simulink model "SimulationLoopNew"  (R2025b)
settings: Solver=VariableStepAuto  StartTime=0.0  StopTime=90  RelTol=1e-3
values from neighbouring files (symbols this model uses):
  dt = 40/10000    (= 0.004)    [constants.m]
  F = StateTransitionMat(z(1:3), z(4:6), R_b2i)    [EstimateStateFCN.m]
  q = q / norm(q)    [EstimateStateFCN.m]
undefined symbols (not defined in the file or in its folder): Checkpoints, constantsASTRA, DiscIntNeverNeededParam, distMode, dt_SIM, HoldTimeReqs, IMU_Rate, K, Light, MIL, u0, x0
libraries: simulink x2, aerolibnav x2, aerolibwind2 x1, dspstat3 x1
settings Model: SimulationMode=accelerator  PacingRate=5  Creator=antho  LastModifiedBy=andrew

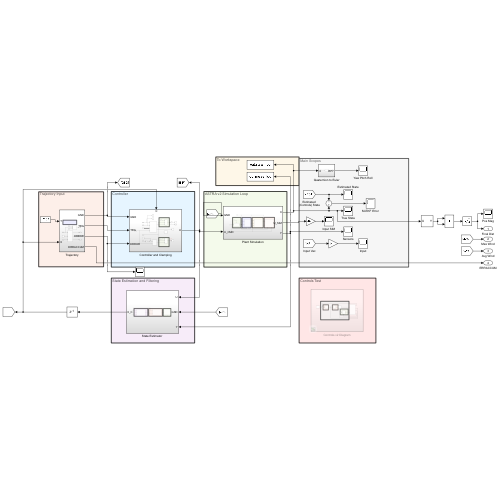
[thumbnail: Simulink's stored preview of the top-level diagram]
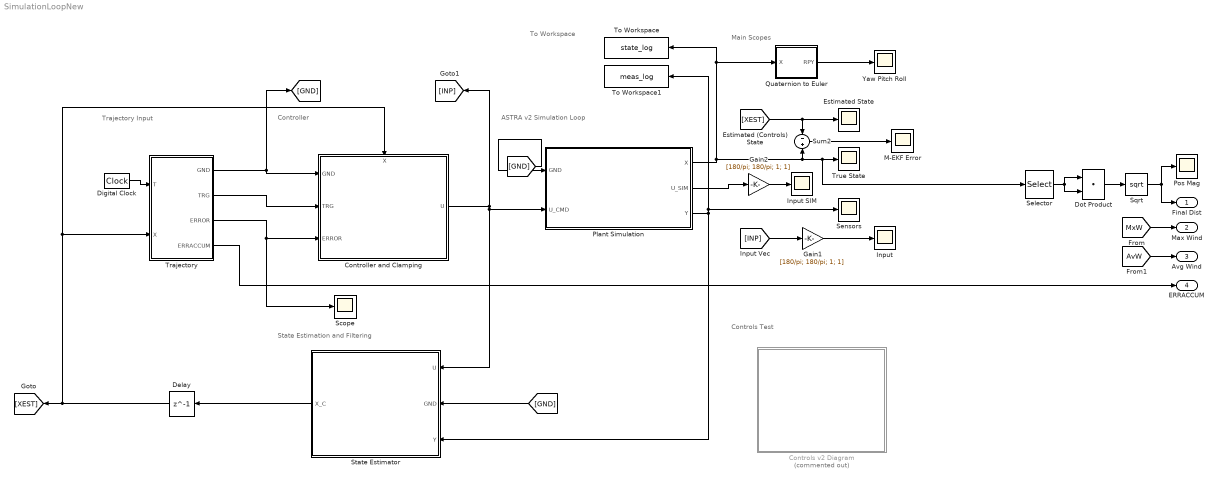
== system SimulationLoopNew ==
  note: To Workspace
  note: Controls Test
  note: Main Scopes
  note: Trajectory Input
  note: State Estimation and Filtering
  note: Controller
  note: ASTRA v2 Simulation Loop
  Controller and Clamping : Subsystem
      settings: PortSchema="{\"entries\":[{\"content\":{\"sides\":[{\"content\":{\"connectorIds\":[\"In1\",\"In2\",\"In3\"]},\"type\":\"ConnectorPlacement.EquallySpacedRectSide\",\"uuid\":\"ecbe546b-cb94-472f-8bff-97599afc2d8a\"},{\"content\":{\"connectorIds\":[\"Out1\"],\"side\":\"RIGHT\"},\"type\":\"ConnectorPlacement.EquallySpacedRectSide\",\"uuid\":\"5863f614-a2a8-49af-9209-63f06ca85da1\"},{\"content\":{\"connectorIds\":[\"In4\"],\"side\":\"TOP\"},\"type\":\"ConnectorPlacement.EquallySpacedRectSide\",\"uuid\":\"6e100a99-a304-4bec-8fe0-0dacf7d0f0e2\"}]},\"type\":\"ConnectorPlacement.EquallySpacedConnector\",\"uuid\":\"0527d0f7-8d45-4b0a-99f9-95f3ca68c54e\"}],\"packageUris\":[\"http://schema.mathworks.com/mf0/Connector/R2020b\"],\"version\":\"1.0\"}"
  Controls v2 Diagram : Subsystem  Commented=on
  Delay : Delay  DelayLength=1  InitialCondition=[1; zeros(15,1)]
  Digital Clock : DigitalClock  SampleTime=dt_SIM
  Dot Product : DotProduct  OutDataTypeStr=Inherit: Inherit via internal rule
  Estimated State : Scope
      settings: ActiveDisplayYMinimum=-0.606468253752392  ActiveDisplayYMaximum=3.4359511007845942
  Gain1 : Gain  Gain=[180/pi; 180/pi; 1; 1]
  Gain2 : Gain  Gain=[180/pi; 180/pi; 1; 1]
  Input : Scope
      settings: ActiveDisplayYMinimum=-12.137518654811966  ActiveDisplayYMaximum=9.237667893307707  DataLoggingVariableName=ScopeData6
  Input SIM : Scope
      settings: ActiveDisplayYMinimum=-12.627100643057217  ActiveDisplayYMaximum=13.453425746992036  DataLoggingVariableName=ScopeData4
  M-EKF Error : Scope
      settings: ActiveDisplayYMinimum=-0.028803808431903943  ActiveDisplayYMaximum=0.022280022235511052  DataLoggingVariableName=ScopeData2
  Plant Simulation : Subsystem
  Pos Mag : Scope
      settings: ActiveDisplayYMinimum=-2.5128820165717731  ActiveDisplayYMaximum=22.615938149145961  DataLoggingVariableName=ScopeData10
  Quaternion to Euler : Subsystem
  Scope : Scope
      settings: ActiveDisplayYMinimum=-6.0728167253221272  ActiveDisplayYMaximum=6.148613432209082  DataLoggingVariableName=ScopeData8
  Selector : Selector  InputPortWidth=16  IndexOptions=Index vector (dialog)  Indices=[5 7]  OutputSizes=1
  Sensors : Scope
      settings: ActiveDisplayYMinimum=-3.2984093858902153  ActiveDisplayYMaximum=20.36574950531497  DataLoggingVariableName=ScopeData3
  Sqrt : Sqrt
  "State Estimator " : Subsystem
  Sum2 : Sum  Inputs=-|+
  To Workspace : ToWorkspace  VariableName=state_log  SaveFormat=Timeseries  SampleTime=-1
  To Workspace1 : ToWorkspace  VariableName=meas_log  SaveFormat=Timeseries  SampleTime=-1
  Trajectory : Subsystem
  True State : Scope
      settings: ActiveDisplayYMinimum=-114.91404993077529  ActiveDisplayYMaximum=77.48765069416325
  Yaw Pitch Roll : Scope
      settings: ActiveDisplayYMinimum=-14.013026351495835  ActiveDisplayYMaximum=17.5900730400627  DataLoggingVariableName=ScopeData7
  Final Dist : Outport
  Max Wind : Outport  Port=2
  Avg Wind : Outport  Port=3
  ERRACCUM : Outport  Port=4
  wires:
  Digital Clock/1 -> Trajectory/1(T)
  "State Estimator "/1(X_C) -> Delay/1
  [XEST] -> Sum2/1, Estimated State/1
  Sum2/1 -> M-EKF Error/1
  Trajectory/3(ERROR) -> Controller and Clamping/3(ERROR), Scope/1
  Controller and Clamping/1(U) -> "State Estimator "/1(U), Plant Simulation/2(U_CMD), [INP]
  Trajectory/1(GND) -> Controller and Clamping/1(GND), [GND]
  [INP] -> Gain1/1
  Gain1/1 -> Input/1
  Delay/1 -> Controller and Clamping/4(X), Trajectory/2(X), [XEST]
  Gain2/1 -> Input SIM/1
  Plant Simulation/2(U_SIM) -> Gain2/1
  Quaternion to Euler/1(RPY) -> Yaw Pitch Roll/1
  [GND] -> Plant Simulation/1(GND)
  [GND] -> "State Estimator "/2(GND)
  Plant Simulation/3(Y) -> To Workspace1/1, Sensors/1, "State Estimator "/3(Y)
  Plant Simulation/1(X) -> Sum2/2, Selector/1, True State/1, Quaternion to Euler/1(X), To Workspace/1
  Trajectory/2(TRG) -> Controller and Clamping/2(TRG)
  Selector/1 -> Dot Product/1, Dot Product/2
  Dot Product/1 -> Sqrt/1
  Sqrt/1 -> Final Dist/1, Pos Mag/1
  [MxW] -> Max Wind/1
  [AvW] -> Avg Wind/1
  Trajectory/4(ERRACCUM) -> ERRACCUM/1

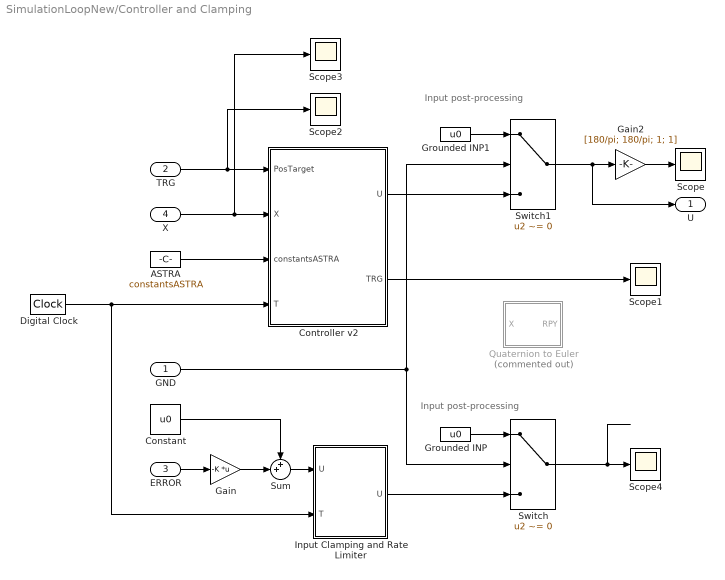
== system SimulationLoopNew/Controller and Clamping ==
  note: Input post-processing
  note: Input post-processing
  GND : Inport
  TRG : Inport  Port=2
  ERROR : Inport  Port=3
  X : Inport  Port=4
  ASTRA : Constant  Value=constantsASTRA  OutDataTypeStr=Bus: slBus1
  Constant : Constant  Value=u0
  Controller v2 : MATLAB Function  TreatAsAtomicUnit=on
  Digital Clock : DigitalClock  SampleTime=dt_SIM
  Gain : Gain  Gain=-K  Multiplication=Matrix(K*u)
  Gain2 : Gain  Gain=[180/pi; 180/pi; 1; 1]
  Grounded INP : Constant  Value=u0
  Grounded INP1 : Constant  Value=u0
  Input Clamping and Rate Limiter : MATLAB Function  TreatAsAtomicUnit=on
  Quaternion to Euler : Subsystem  Commented=on
  Scope{,1..4} (5 alike) : Scope
      Scope settings: ActiveDisplayYMinimum=-11.801195540279929  ActiveDisplayYMaximum=6.2107598625193638  DataLoggingVariableName=ScopeData9
      Scope1 settings: ActiveDisplayYMinimum=-1.875  ActiveDisplayYMaximum=1.875  DataLoggingVariableName=ScopeData17
      Scope2 settings: ActiveDisplayYMinimum=-1  ActiveDisplayYMaximum=1  DataLoggingVariableName=ScopeData18
      Scope3 settings: ActiveDisplayYMinimum=-0.53566092037557744  ActiveDisplayYMaximum=3.4212061004598149  DataLoggingVariableName=ScopeData19
      Scope4 settings: ActiveDisplayYMinimum=-5.4940505752964679  ActiveDisplayYMaximum=15.32295755496437  DataLoggingVariableName=ScopeData20
  Sum : Sum  Inputs=++|
  Switch : Switch  Criteria=u2 ~= 0  SaturateOnIntegerOverflow=off  InputSameDT=off
  Switch1 : Switch  Criteria=u2 ~= 0  SaturateOnIntegerOverflow=off  InputSameDT=off
  U : Outport
  wires:
  ERROR/1 -> Gain/1
  Digital Clock/1 -> Controller v2/4(T), Input Clamping and Rate Limiter/2(T)
  Input Clamping and Rate Limiter/1(U) -> Switch/3
  Switch/1 -> Scope4/1
  Grounded INP/1 -> Switch/1
  Sum/1 -> Input Clamping and Rate Limiter/1("U ")
  Gain/1 -> Sum/2
  Constant/1 -> Sum/1
  Controller v2/1(U) -> Switch1/3
  GND/1 -> Switch1/2, Switch/2
  Grounded INP1/1 -> Switch1/1
  Switch1/1 -> U/1, Gain2/1
  TRG/1 -> Scope2/1, Controller v2/1(PosTarget)
  X/1 -> Scope3/1, Controller v2/2(X)
  ASTRA/1 -> Controller v2/3(constantsASTRA)
  Gain2/1 -> Scope/1
  Controller v2/2(TRG) -> Scope1/1

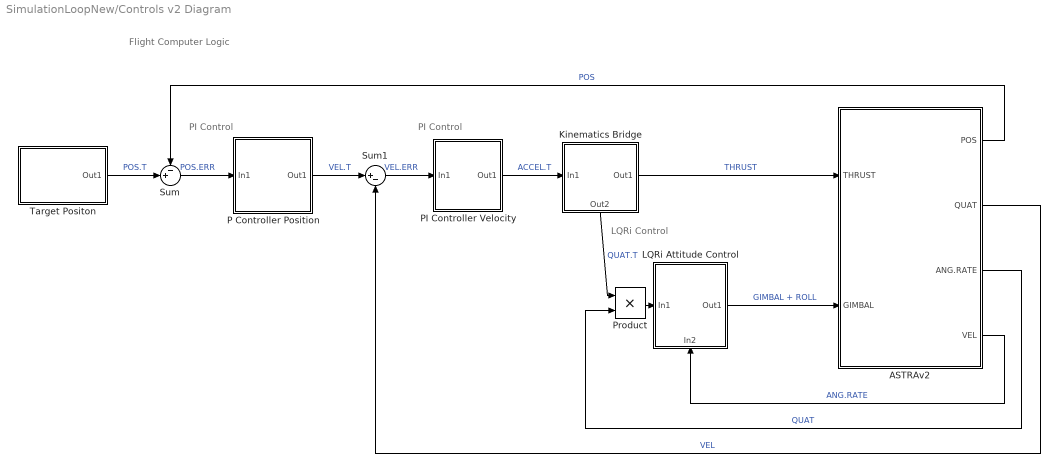
== system SimulationLoopNew/Controls v2 Diagram ==
  note: PI Control
  note: Flight Computer Logic
  note: PI Control
  note: LQRi Control
  ASTRAv2 : Subsystem
  Kinematics Bridge : Subsystem
      settings: PortSchema="{\"entries\":[{\"content\":{\"sides\":[{\"content\":{\"connectorIds\":[\"In1\"]},\"type\":\"ConnectorPlacement.EquallySpacedRectSide\",\"uuid\":\"14f1819f-c5b0-4857-8a3f-059930327852\"},{\"content\":{\"connectorIds\":[\"Out1\"],\"side\":\"RIGHT\"},\"type\":\"ConnectorPlacement.EquallySpacedRectSide\",\"uuid\":\"f1c93ae3-8d17-4b74-967d-9d6328e115fb\"},{\"content\":{\"side\":\"TOP\"},\"type\":\"ConnectorPlacement.EquallySpacedRectSide\",\"uuid\":\"bc82f49d-1f27-4136-b175-63a6ad0dbf5b\"},{\"content\":{\"connectorIds\":[\"Out2\"],\"side\":\"BOTTOM\"},\"type\":\"ConnectorPlacement.EquallySpacedRectSide\",\"uuid\":\"6dcf9527-a6d9-4dea-a2bb-d98c67e6f046\"}]},\"type\":\"ConnectorPlacement.EquallySpacedConnector\",\"uuid\":\"f166f20b-cbf6-467f-83b3-19efe4727134\"}],\"packageUris\":[\"http://schema.mathworks.com/mf0/Connector/R2020b\"],\"version\":\"1.0\"}"
  LQRi Attitude Control : Subsystem
      settings: PortSchema="{\"entries\":[{\"content\":{\"sides\":[{\"content\":{\"connectorIds\":[\"In1\"]},\"type\":\"ConnectorPlacement.EquallySpacedRectSide\",\"uuid\":\"cd9cee5f-4e02-4c25-b158-b6d381dcbc8d\"},{\"content\":{\"connectorIds\":[\"Out1\"],\"side\":\"RIGHT\"},\"type\":\"ConnectorPlacement.EquallySpacedRectSide\",\"uuid\":\"2ef087dd-7fcc-4555-b2da-05ccf598bd0a\"},{\"content\":{\"side\":\"TOP\"},\"type\":\"ConnectorPlacement.EquallySpacedRectSide\",\"uuid\":\"5427ed8c-500e-4860-8e5f-93d13574dd24\"},{\"content\":{\"connectorIds\":[\"In2\"],\"side\":\"BOTTOM\"},\"type\":\"ConnectorPlacement.EquallySpacedRectSide\",\"uuid\":\"f48b80df-9658-4fd9-b967-6adbaff8a875\"}]},\"type\":\"ConnectorPlacement.EquallySpacedConnector\",\"uuid\":\"547d8ec4-1c4e-4f3b-85b8-72bd650a229d\"}],\"packageUris\":[\"http://schema.mathworks.com/mf0/Connector/R2020b\"],\"version\":\"1.0\"}"
  P Controller Position : Subsystem
  PI Controller Velocity : Subsystem
  Product : Product
  Sum : Sum  Inputs=-+|
  Sum1 : Sum  Inputs=|+-
  Target Positon : Subsystem
  wires:
  P Controller Position/1(Out1) -> Sum1/1  "VEL.T"
  Sum1/1 -> PI Controller Velocity/1(In1)  "VEL.ERR"
  PI Controller Velocity/1(Out1) -> Kinematics Bridge/1(In1)  "ACCEL.T"
  Sum/1 -> P Controller Position/1(In1)  "POS.ERR"
  Kinematics Bridge/2(Out2) -> Product/1  "QUAT.T"
  Product/1 -> LQRi Attitude Control/1(In1)
  LQRi Attitude Control/1(Out1) -> ASTRAv2/2("GIMBAL ")  "GIMBAL + ROLL"
  Kinematics Bridge/1(Out1) -> ASTRAv2/1(THRUST)  "THRUST"
  Target Positon/1(Out1) -> Sum/2  "POS.T"
  ASTRAv2/1(POS) -> Sum/1  "POS"
  ASTRAv2/2(QUAT) -> Sum1/2  "VEL"
  ASTRAv2/3(ANG.RATE) -> Product/2  "QUAT"
  ASTRAv2/4(VEL) -> LQRi Attitude Control/2(In2)  "ANG.RATE"

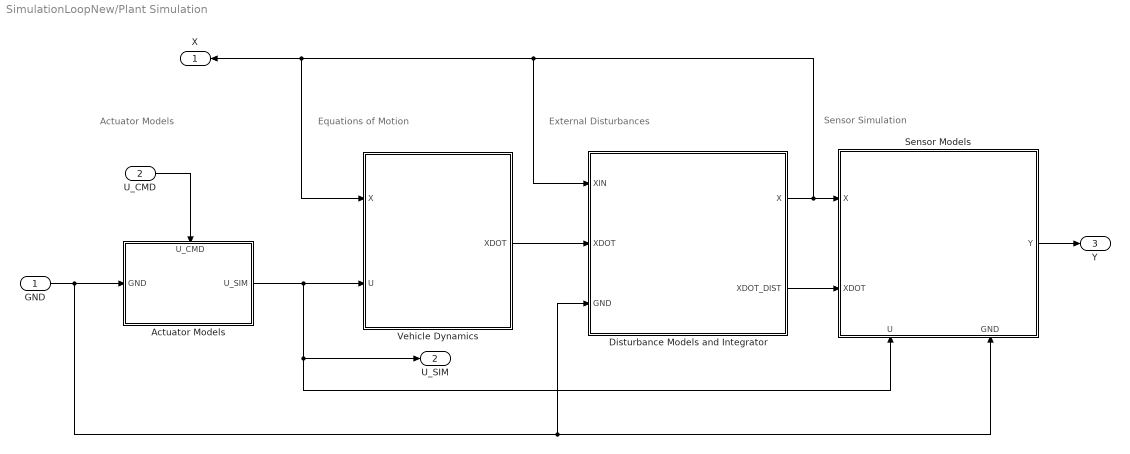
== system SimulationLoopNew/Plant Simulation ==
  note: Equations of Motion
  note: Actuator Models
  note: External Disturbances
  note: Sensor Simulation
  GND : Inport
  U_CMD : Inport  Port=2
  Actuator Models : Subsystem
      settings: PortSchema="{\"entries\":[{\"content\":{\"sides\":[{\"content\":{\"connectorIds\":[\"In1\"]},\"type\":\"ConnectorPlacement.EquallySpacedRectSide\",\"uuid\":\"54343072-6023-41e9-a0f6-81f6bed17e05\"},{\"content\":{\"connectorIds\":[\"Out1\"],\"side\":\"RIGHT\"},\"type\":\"ConnectorPlacement.EquallySpacedRectSide\",\"uuid\":\"2ed3290f-d38b-41d8-95ae-d88068502334\"},{\"content\":{\"connectorIds\":[\"In2\"],\"side\":\"TOP\"},\"type\":\"ConnectorPlacement.EquallySpacedRectSide\",\"uuid\":\"e9e41c57-b871-4be2-92e8-dfbbf995d6b0\"}]},\"type\":\"ConnectorPlacement.EquallySpacedConnector\",\"uuid\":\"c037521e-b20b-40c6-bb74-3aafe8fc1476\"}],\"packageUris\":[\"http://schema.mathworks.com/mf0/Connector/R2020b\"],\"version\":\"1.0\"}"
  Disturbance Models and Integrator : Subsystem
  Sensor Models : Subsystem
      settings: PortSchema="{\"entries\":[{\"content\":{\"sides\":[{\"content\":{\"connectorIds\":[\"In1\",\"In2\"]},\"type\":\"ConnectorPlacement.EquallySpacedRectSide\",\"uuid\":\"9bc4a206-bba4-4c50-88a9-89b0392ab722\"},{\"content\":{\"connectorIds\":[\"Out1\"],\"side\":\"RIGHT\"},\"type\":\"ConnectorPlacement.EquallySpacedRectSide\",\"uuid\":\"162bbd17-e1b8-4f29-9191-53e17e38d79d\"},{\"content\":{\"side\":\"TOP\"},\"type\":\"ConnectorPlacement.EquallySpacedRectSide\",\"uuid\":\"c56a23db-6a5c-435f-99fd-d50fc9dbdc94\"},{\"content\":{\"connectorIds\":[\"In3\",\"In4\"],\"side\":\"BOTTOM\"},\"type\":\"ConnectorPlacement.EquallySpacedRectSide\",\"uuid\":\"e0c2a0dc-3b7a-40ac-8345-28e7bf7b9405\"}]},\"type\":\"ConnectorPlacement.EquallySpacedConnector\",\"uuid\":\"d1c29f55-9be5-4f45-9d70-06beba2c2f44\"}],\"packageUris\":[\"http://schema.mathworks.com/mf0/Connector/R2020b\"],\"version\":\"1.0\"}"
  Vehicle Dynamics : Subsystem
  X : Outport
  U_SIM : Outport  Port=2
  Y : Outport  Port=3
  wires:
  U_CMD/1 -> Actuator Models/2(U_CMD)
  Vehicle Dynamics/1(XDOT) -> Disturbance Models and Integrator/2(XDOT)
  Sensor Models/1(Y) -> Y/1
  GND/1 -> Actuator Models/1(GND), Sensor Models/4(GND), Disturbance Models and Integrator/3(GND)
  Disturbance Models and Integrator/1(X) -> Disturbance Models and Integrator/1(XIN), Vehicle Dynamics/1(X), X/1, Sensor Models/1(X)
  Disturbance Models and Integrator/2(XDOT_DIST) -> Sensor Models/2(XDOT)
  Actuator Models/1(U_SIM) -> U_SIM/1, Sensor Models/3(U), Vehicle Dynamics/2(U)

== system SimulationLoopNew/Quaternion to Euler ==
  X : Inport
  Quaternion to Euler : MATLAB Function  TreatAsAtomicUnit=on
  RPY : Outport
  wires:
  X/1 -> Quaternion to Euler/1(X)
  Quaternion to Euler/1(Angles) -> RPY/1

== system SimulationLoopNew/State Estimator  ==
  note: Sequential Notch Filter for IMU
  note: State Augmentator
  note: Kalman Filtering
  U : Inport
  GND : Inport  Port=2
  Y : Inport  Port=3
  Adaptive Notch Filter [ANF] : Subsystem
  Multiplicative Extended Kalman Filter [M-EKF] : Subsystem
  State Augmentator : Subsystem
      settings: PortSchema="{\"entries\":[{\"content\":{\"sides\":[{\"content\":{\"connectorIds\":[\"In1\"]},\"type\":\"ConnectorPlacement.EquallySpacedRectSide\",\"uuid\":\"bb6458aa-622a-4d42-b468-f616d6e302fe\"},{\"content\":{\"connectorIds\":[\"Out1\"],\"side\":\"RIGHT\"},\"type\":\"ConnectorPlacement.EquallySpacedRectSide\",\"uuid\":\"af8bade2-eb0a-4714-9db5-d33244eb3558\"},{\"content\":{\"side\":\"TOP\"},\"type\":\"ConnectorPlacement.EquallySpacedRectSide\",\"uuid\":\"05a7f106-e447-475e-b3b5-727cb0579a7b\"},{\"content\":{\"connectorIds\":[\"In2\"],\"side\":\"BOTTOM\"},\"type\":\"ConnectorPlacement.EquallySpacedRectSide\",\"uuid\":\"a6d44455-a42d-44f7-b37b-0d3db398c8f2\"}]},\"type\":\"ConnectorPlacement.EquallySpacedConnector\",\"uuid\":\"c6f62579-6b17-43b5-92f1-6190f0d9fd8b\"}],\"packageUris\":[\"http://schema.mathworks.com/mf0/Connector/R2020b\"],\"version\":\"1.0\"}"
  X_C : Outport
  wires:
  Multiplicative Extended Kalman Filter [M-EKF]/1(X) -> State Augmentator/1(X_KF)
  State Augmentator/1(X) -> X_C/1
  Adaptive Notch Filter [ANF]/1(Y_FILT) -> State Augmentator/2(Y.FILT), Multiplicative Extended Kalman Filter [M-EKF]/2(Y)
  GND/1 -> Adaptive Notch Filter [ANF]/1(GND), Multiplicative Extended Kalman Filter [M-EKF]/1(GND)
  Y/1 -> Adaptive Notch Filter [ANF]/3(Y)
  U/1 -> Adaptive Notch Filter [ANF]/2(U)

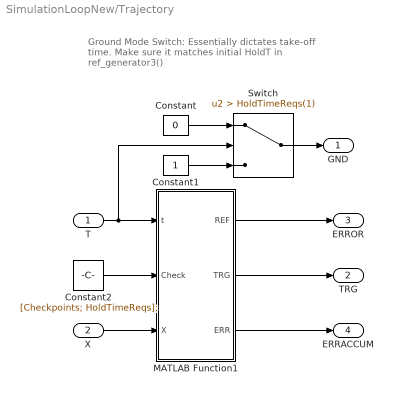
== system SimulationLoopNew/Trajectory ==
  note: Ground Mode Switch:
      | Essentially dictates take-off time.
      | Make sure it matches initial HoldT
      | in ref_generator3()
  T : Inport
  X : Inport  Port=2
  Constant : Constant  Value=0
  Constant1 : Constant
  Constant2 : Constant  Value=[Checkpoints; HoldTimeReqs];
  MATLAB Function1 : MATLAB Function  TreatAsAtomicUnit=on
  Switch : Switch  Criteria=u2 > Threshold  Threshold=HoldTimeReqs(1)  SaturateOnIntegerOverflow=off  InputSameDT=off
  GND : Outport
  TRG : Outport  Port=2
  ERROR : Outport  Port=3
  ERRACCUM : Outport  Port=4
  wires:
  T/1 -> Switch/2, MATLAB Function1/1(t)
  X/1 -> MATLAB Function1/3(X)
  MATLAB Function1/1(REF) -> ERROR/1
  Constant/1 -> Switch/1
  Constant1/1 -> Switch/3
  Switch/1 -> GND/1
  Constant2/1 -> MATLAB Function1/2(Check)
  MATLAB Function1/2(TRG) -> TRG/1
  MATLAB Function1/3(ERR) -> ERRACCUM/1

== system SimulationLoopNew/Controller and Clamping/Quaternion to Euler ==
  X : Inport
  Quaternion to Euler : MATLAB Function  TreatAsAtomicUnit=on
  RPY : Outport
  wires:
  X/1 -> Quaternion to Euler/1(X)
  Quaternion to Euler/1(Angles) -> RPY/1

== system SimulationLoopNew/Controls v2 Diagram/ASTRAv2 ==
  THRUST : Inport
  "GIMBAL " : Inport  Port=2
  POS : Outport
  QUAT : Outport  Port=2
  ANG.RATE : Outport  Port=3
  VEL : Outport  Port=4
  wires:
  THRUST/1 -> POS/1

== system SimulationLoopNew/Controls v2 Diagram/Kinematics Bridge ==
  In1 : Inport
  Out1 : Outport
  Out2 : Outport  Port=2
  wires:
  In1/1 -> Out2/1, Out1/1

== system SimulationLoopNew/Controls v2 Diagram/LQRi Attitude Control ==
  In1 : Inport
  In2 : Inport  Port=2
  Out1 : Outport
  wires:
  In1/1 -> Out1/1

== system SimulationLoopNew/Controls v2 Diagram/P Controller Position ==
  In1 : Inport
  Out1 : Outport
  wires:
  In1/1 -> Out1/1

== system SimulationLoopNew/Controls v2 Diagram/PI Controller Velocity ==
  In1 : Inport
  Out1 : Outport
  wires:
  In1/1 -> Out1/1

== system SimulationLoopNew/Controls v2 Diagram/Target Positon ==
  Out1 : Outport
  wires:
  ? -> Out1/1

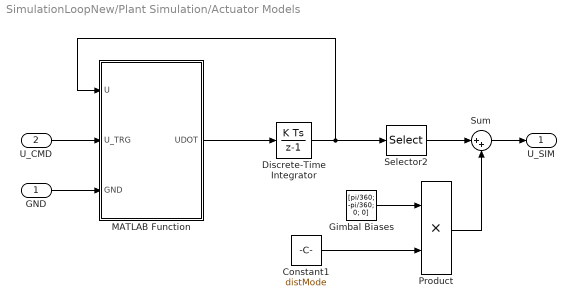
== system SimulationLoopNew/Plant Simulation/Actuator Models ==
  GND : Inport
  U_CMD : Inport  Port=2
  Constant1 : Constant  Value=distMode
  Discrete-Time Integrator : DiscreteIntegrator  InitialCondition=[zeros(4,1); u0(3); 0]  SampleTime=-1  ICPrevOutput=DiscIntNeverNeededParam  ICPrevScaledInput=DiscIntNeverNeededParam
  Gimbal Biases : Constant  Value=[pi/360; -pi/360; 0; 0]
  MATLAB Function : MATLAB Function  TreatAsAtomicUnit=on
  Product : Product
  Selector2 : Selector  InputPortWidth=6  IndexOptions=Index vector (dialog)  Indices=[1 3 5 6]  OutputSizes=1
  Sum : Sum  Inputs=|++
  U_SIM : Outport
  wires:
  U_CMD/1 -> MATLAB Function/2(U_TRG)
  MATLAB Function/1(UDOT) -> Discrete-Time Integrator/1
  Discrete-Time Integrator/1 -> MATLAB Function/1(U), Selector2/1
  GND/1 -> MATLAB Function/3(GND)
  Sum/1 -> U_SIM/1
  Selector2/1 -> Sum/1
  Gimbal Biases/1 -> Product/1
  Product/1 -> Sum/2
  Constant1/1 -> Product/2

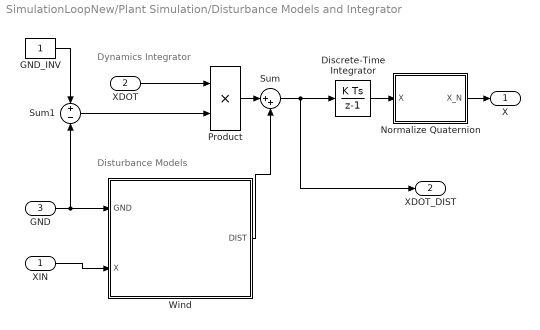
== system SimulationLoopNew/Plant Simulation/Disturbance Models and Integrator ==
  note: Disturbance Models
  note: Dynamics Integrator
  XIN : Inport
  XDOT : Inport  Port=2
  GND : Inport  Port=3
  Discrete-Time Integrator : DiscreteIntegrator  InitialCondition=x0  SampleTime=-1  ICPrevOutput=DiscIntNeverNeededParam  ICPrevScaledInput=DiscIntNeverNeededParam
  GND_INV : Constant
  Normalize Quaternion : MATLAB Function  TreatAsAtomicUnit=on
  Product : Product
  Sum : Sum  Inputs=|++
  Sum1 : Sum  Inputs=+|-
  Wind : Subsystem
  X : Outport
  XDOT_DIST : Outport  Port=2
  wires:
  Discrete-Time Integrator/1 -> Normalize Quaternion/1(X)
  XIN/1 -> Wind/2(X)
  Wind/1(DIST) -> Sum/2
  XDOT/1 -> Product/1
  GND_INV/1 -> Sum1/1
  Sum1/1 -> Product/2
  GND/1 -> Wind/1(GND), Sum1/2
  Product/1 -> Sum/1
  Sum/1 -> Discrete-Time Integrator/1, XDOT_DIST/1
  Normalize Quaternion/1(X_N) -> X/1

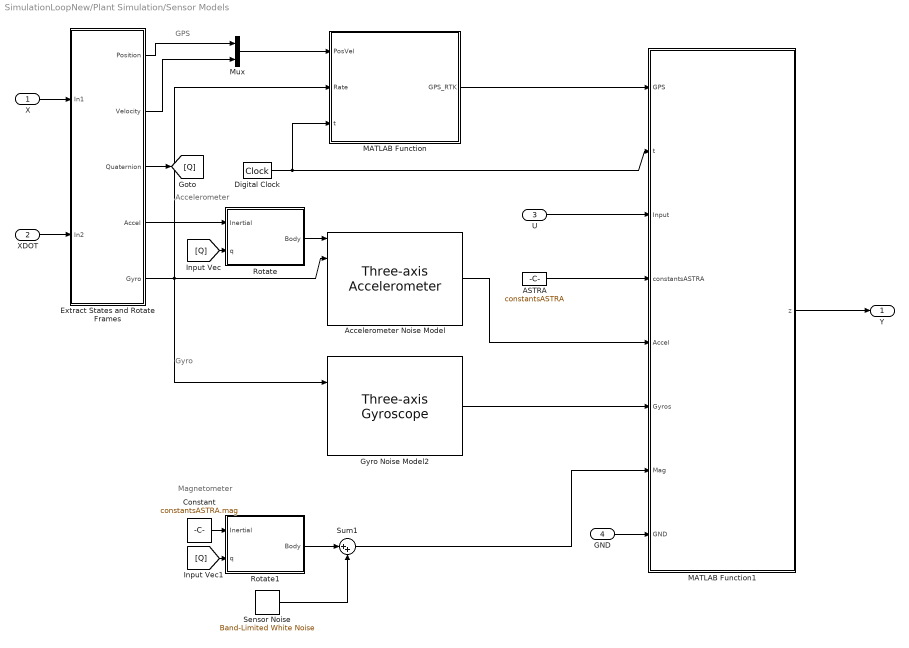
== system SimulationLoopNew/Plant Simulation/Sensor Models ==
  note: Gyro
  note: Accelerometer
  note: Magnetometer
  note: GPS
  X : Inport
  XDOT : Inport  Port=2
  U : Inport  Port=3
  GND : Inport  Port=4
  ASTRA : Constant  Value=constantsASTRA  OutDataTypeStr=Bus: slBus1
  Accelerometer Noise Model : aerolibnav/Three-axis Accelerometer  units=Metric (MKS)  acc=[0 0 0.15]  gtype=on  dtype_a=on  w_a=190  z_a=0.707  a_sf_cc=eye(3)  a_bias=[0.09, 0.09, 0.09]  a_Ts=1 / IMU_Rate  a_rand=on  a_seeds=[23093 23094 23095]  a_pow=ones(1,3) * 0.008^2 * 1 / IMU_Rate  a_sat="[-inf  -inf  -inf  inf inf inf]"
  Constant : Constant  Value=constantsASTRA.mag
  Digital Clock : DigitalClock  SampleTime=dt_SIM
  Extract States and Rotate Frames : Subsystem
  Gyro Noise Model2 : aerolibnav/Three-axis Gyroscope  dtype_g=on  w_g=190  z_g=0.707  g_sf_cc=eye(3)  g_bias=0.005 * ones(1,3)  g_sen=0  g_Ts=1 / IMU_Rate  g_rand=on  g_seeds=[23093 23094 23095]  g_pow=ones(1,3) * 0.003^2 * dt  g_sat="[-inf  -inf  -inf  inf inf inf]"
  MATLAB Function : MATLAB Function  TreatAsAtomicUnit=on
  MATLAB Function1 : MATLAB Function  TreatAsAtomicUnit=on
  Mux : Mux  Inputs=2
  Rotate : MATLAB Function  TreatAsAtomicUnit=on
  Rotate1 : MATLAB Function  TreatAsAtomicUnit=on
  Sensor Noise : simulink/Sources/Band-Limited White Noise  Cov=(4E-4)^2  Ts=dt_SIM  seed=[23341,23342,23343]
  Sum1 : Sum  Inputs=|++
  Y : Outport
  wires:
  X/1 -> Extract States and Rotate Frames/1(In1)
  XDOT/1 -> Extract States and Rotate Frames/2(In2)
  Digital Clock/1 -> MATLAB Function/3(t), MATLAB Function1/2(t)
  Extract States and Rotate Frames/5(Gyro) -> Accelerometer Noise Model/2, Gyro Noise Model2/1, MATLAB Function/2(Rate)
  Extract States and Rotate Frames/3(Quaternion) -> [Q]
  Rotate/1(Body) -> Accelerometer Noise Model/1
  Extract States and Rotate Frames/4(Accel) -> Rotate/1(Inertial)
  [Q] -> Rotate/2(q)
  Constant/1 -> Rotate1/1(Inertial)
  [Q] -> Rotate1/2(q)
  Sensor Noise/1 -> Sum1/2
  Rotate1/1(Body) -> Sum1/1
  Sum1/1 -> MATLAB Function1/7(Mag)
  MATLAB Function/1(GPS_RTK) -> MATLAB Function1/1(GPS)
  Accelerometer Noise Model/1 -> MATLAB Function1/5(Accel)
  Gyro Noise Model2/1 -> MATLAB Function1/6(Gyros)
  MATLAB Function1/1(z) -> Y/1
  ASTRA/1 -> MATLAB Function1/4(constantsASTRA)
  Extract States and Rotate Frames/2(Velocity) -> Mux/2
  Mux/1 -> MATLAB Function/1(PosVel)
  Extract States and Rotate Frames/1(Position) -> Mux/1
  U/1 -> MATLAB Function1/3(Input)
  GND/1 -> MATLAB Function1/8(GND)

== system SimulationLoopNew/Plant Simulation/Vehicle Dynamics ==
  X : Inport
  U : Inport  Port=2
  Constant : Constant  Value=distMode
  Dynamics : MATLAB Function  TreatAsAtomicUnit=on
  XDOT : Outport
  wires:
  Dynamics/1(XDOT) -> XDOT/1
  U/1 -> Dynamics/2(U)
  X/1 -> Dynamics/1(X)
  Constant/1 -> Dynamics/3(distMode)

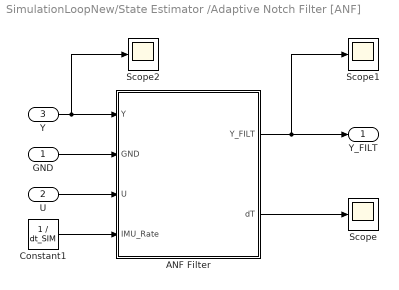
== system SimulationLoopNew/State Estimator /Adaptive Notch Filter [ANF] ==
  GND : Inport
  U : Inport  Port=2
  Y : Inport  Port=3
  ANF Filter : MATLAB Function  TreatAsAtomicUnit=on
  Constant1 : Constant  Value=1 / dt_SIM
  Scope : Scope
      settings: ActiveDisplayYMinimum=0.00097880622837365075  ActiveDisplayYMaximum=0.0020384948096911198  DataLoggingVariableName=ScopeData12
  Scope1 : Scope
      settings: ActiveDisplayYMinimum=-3.6072966974512437  ActiveDisplayYMaximum=13.831448470901217  DataLoggingVariableName=ScopeData15
  Scope2 : Scope
      settings: ActiveDisplayYMinimum=-0.822722965610661  ActiveDisplayYMaximum=0.985135629551039  DataLoggingVariableName=ScopeData16
  Y_FILT : Outport
  wires:
  ANF Filter/1(Y_FILT) -> Scope1/1, Y_FILT/1
  GND/1 -> ANF Filter/2(GND)
  U/1 -> ANF Filter/3(U)
  Y/1 -> Scope2/1, ANF Filter/1(Y)
  Constant1/1 -> ANF Filter/4(IMU_Rate)
  ANF Filter/2(dT) -> Scope/1

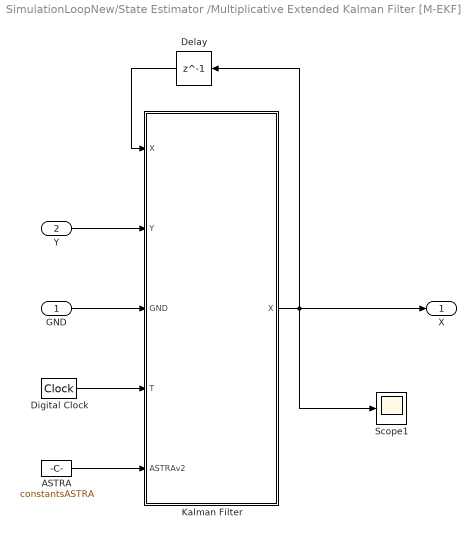
== system SimulationLoopNew/State Estimator /Multiplicative Extended Kalman Filter [M-EKF] ==
  GND : Inport
  Y : Inport  Port=2
  ASTRA : Constant  Value=constantsASTRA  OutDataTypeStr=Bus: slBus1
  Delay : Delay  DelayLength=1  InitialCondition=[1; zeros(18,1)]
  Digital Clock : DigitalClock  SampleTime=dt_SIM
  Kalman Filter : MATLAB Function  TreatAsAtomicUnit=on
  Scope1 : Scope
      settings: ActiveDisplayYMinimum=-0.76732597177813688  ActiveDisplayYMaximum=3.5267061535948003  DataLoggingVariableName=ScopeData11
  X : Outport
  wires:
  Digital Clock/1 -> Kalman Filter/4(T)
  Kalman Filter/1(X) -> Delay/1, X/1, Scope1/1
  Y/1 -> Kalman Filter/2(Y)
  Delay/1 -> Kalman Filter/1("X ")
  ASTRA/1 -> Kalman Filter/5(ASTRAv2)
  GND/1 -> Kalman Filter/3(GND)

== system SimulationLoopNew/State Estimator /State Augmentator ==
  X_KF : Inport
  Y.FILT : Inport  Port=2
  MATLAB Function : MATLAB Function  TreatAsAtomicUnit=on
  X : Outport
  wires:
  X_KF/1 -> MATLAB Function/1(XKF)
  MATLAB Function/1(X) -> X/1
  Y.FILT/1 -> MATLAB Function/2(Y)

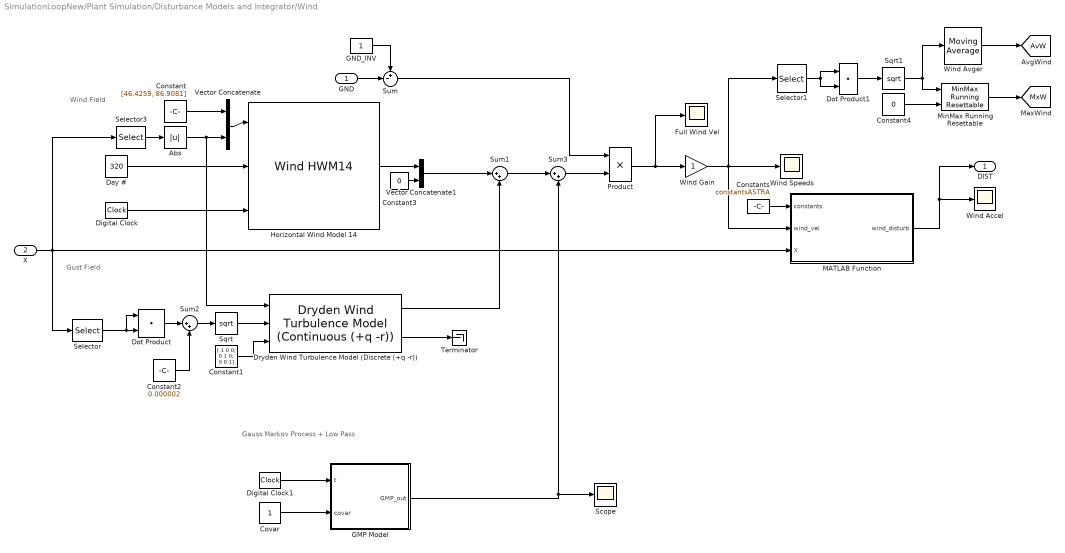
== system SimulationLoopNew/Plant Simulation/Disturbance Models and Integrator/Wind ==
  note: Gauss Markov Process + Low Pass
  note: Gust Field
  note: Wind Field
  GND : Inport
  X : Inport  Port=2
  Abs : Abs  SaturateOnIntegerOverflow=off
  Constant : Constant  Value=[46.4259, 86.9081]
  Constant1 : Constant  Value=[-1 0 0; 0 1 0; 0 0 1]
  Constant2 : Constant  Value=0.000002
  Constant3 : Constant  Value=0
  Constant4 : Constant  Value=0
  Constants : Constant  Value=constantsASTRA  OutDataTypeStr=Bus: slBus1
  Covar : Constant
  Day # : Constant  Value=320
  Digital Clock : DigitalClock  SampleTime=dt_SIM
  Digital Clock1 : DigitalClock  SampleTime=dt_SIM
  Dot Product : DotProduct  OutDataTypeStr=Inherit: Inherit via internal rule
  Dot Product1 : DotProduct  OutDataTypeStr=Inherit: Inherit via internal rule
  Dryden Wind Turbulence Model (Discrete (+q -r)) : aerolibwind2/Dryden Wind Turbulence Model  (Continuous (+q -r))  units=Metric (MKS)  spec=MIL-F-8785C  model=Discrete Dryden (+q -r)  W20=15  Wdeg=0  TurbProb=10^-2 - Light  L_high=533.4  Wingspan=10  ts=0.1  Seed=[23341 23342 23343 23344]  T_on=on
      settings: LibrarySourceBlock=|
      | aerolibwind2/Dryden Wind Turbulence Model
      | (Discrete (+q -r))
  Full Wind Vel : Scope
      settings: ActiveDisplayYMinimum=-3.7865155465706426  ActiveDisplayYMaximum=6.511644105884  DataLoggingVariableName=ScopeData13
  GMP Model : MATLAB Function  TreatAsAtomicUnit=on
  GND_INV : Constant
  Horizontal Wind Model 14 : WindHWM14
  MATLAB Function : MATLAB Function  TreatAsAtomicUnit=on
  MinMax Running Resettable : simulink/Math Operations/MinMax Running Resettable  Function=max  vinit=0.0
  Product : Product
  Scope : Scope
      settings: ActiveDisplayYMinimum=-2.8676060433464485  ActiveDisplayYMaximum=2.8612107779538238  DataLoggingVariableName=ScopeData14
  Selector : Selector  InputPortWidth=16  IndexOptions=Index vector (dialog)  Indices=[8:10]  OutputSizes=1
  Selector1 : Selector  InputPortWidth=3  IndexOptions=Index vector (dialog)  Indices=[1 3]  OutputSizes=1
  Selector3 : Selector  InputPortWidth=16  IndexOptions=Index vector (dialog)  Indices=7  OutputSizes=1
  Sqrt : Sqrt
  Sqrt1 : Sqrt
  Sum : Sum  Inputs=+-|
  Sum1 : Sum  Inputs=|++
  Sum2 : Sum  Inputs=|++
  Sum3 : Sum  Inputs=|++
  Terminator : Terminator
  Vector Concatenate : Concatenate
  Vector Concatenate1 : Concatenate
  Wind Accel : Scope
      settings: ActiveDisplayYMinimum=-4.309101340154939  ActiveDisplayYMaximum=3.0691763455484393  DataLoggingVariableName=ScopeData5
  Wind Avger : dspstat3/Moving Average  Method=Sliding window  ForgettingFactorPort=off  SpecifyWindowLength=off  WindowLength=4  OverlapLength=3  AllowArbitraryInputLength=off  ForgettingFactor=0.9  SimulateUsing=Interpreted execution
  Wind Gain : Gain
  Wind Speeds : Scope
      settings: ActiveDisplayYMinimum=-7.0438056350535074  ActiveDisplayYMaximum=6.4425491694674681  DataLoggingVariableName=ScopeData5
  DIST : Outport
  tag scope: AvW=global, MxW=global
  wires:
  Digital Clock/1 -> Horizontal Wind Model 14/3
  Day #/1 -> Horizontal Wind Model 14/2
  MATLAB Function/1(wind_disturb) -> DIST/1, Wind Accel/1
  Vector Concatenate/1 -> Horizontal Wind Model 14/1
  Selector3/1 -> Abs/1
  Constant/1 -> Vector Concatenate/1
  GND/1 -> Sum/2
  Sum/1 -> Product/1
  GND_INV/1 -> Sum/1
  Horizontal Wind Model 14/1 -> Vector Concatenate1/1
  Constants/1 -> MATLAB Function/1(constants)
  Selector/1 -> Dot Product/1, Dot Product/2
  Sqrt/1 -> Dryden Wind Turbulence Model (Discrete (+q -r))/2
  Dryden Wind Turbulence Model (Discrete (+q -r))/1 -> Sum1/2
  Constant1/1 -> Dryden Wind Turbulence Model (Discrete (+q -r))/3
  Sum2/1 -> Sqrt/1
  Dot Product/1 -> Sum2/1
  Constant2/1 -> Sum2/2
  X/1 -> Selector3/1, MATLAB Function/3(X), Selector/1
  Abs/1 -> Dryden Wind Turbulence Model (Discrete (+q -r))/1, Vector Concatenate/2
  Product/1 -> Full Wind Vel/1, Wind Gain/1
  Vector Concatenate1/1 -> Sum1/1
  Constant3/1 -> Vector Concatenate1/2
  Dryden Wind Turbulence Model (Discrete (+q -r))/2 -> Terminator/1
  Wind Gain/1 -> Selector1/1, Wind Speeds/1, MATLAB Function/2(wind_vel)
  Sum3/1 -> Product/2
  Sum1/1 -> Sum3/1
  GMP Model/1(GMP_out) -> Scope/1, Sum3/2
  Digital Clock1/1 -> GMP Model/1(t)
  Selector1/1 -> Dot Product1/1, Dot Product1/2
  Dot Product1/1 -> Sqrt1/1
  Constant4/1 -> MinMax Running Resettable/2
  Sqrt1/1 -> Wind Avger/1, MinMax Running Resettable/1
  Wind Avger/1 -> [AvW]
  MinMax Running Resettable/1 -> [MxW]
  Covar/1 -> GMP Model/2(covar)

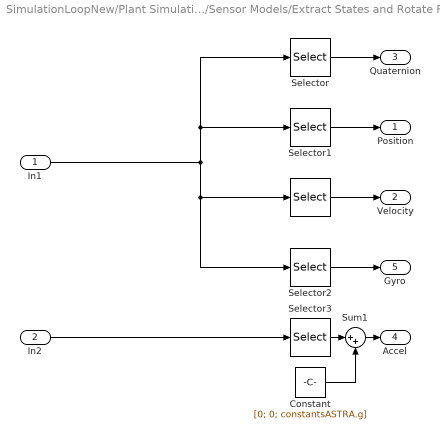
== system SimulationLoopNew/Plant Simulation/Sensor Models/Extract States and Rotate Frames ==
  In1 : Inport
  In2 : Inport  Port=2
  "  " : Selector  InputPortWidth=16  IndexOptions=Index vector (dialog)  Indices=[8:10]  OutputSizes=1
  Constant : Constant  Value=[0; 0; constantsASTRA.g]
  Selector : Selector  InputPortWidth=16  IndexOptions=Index vector (dialog)  Indices=[1:4]  OutputSizes=1
  Selector1 : Selector  InputPortWidth=16  IndexOptions=Index vector (dialog)  Indices=[5:7]  OutputSizes=1
  Selector2 : Selector  InputPortWidth=16  IndexOptions=Index vector (dialog)  Indices=[11:13]  OutputSizes=1
  Selector3 : Selector  InputPortWidth=16  IndexOptions=Index vector (dialog)  Indices=[8:10]  OutputSizes=1
  Sum1 : Sum  Inputs=|++
  Position : Outport
  Velocity : Outport  Port=2
  Quaternion : Outport  Port=3
  Accel : Outport  Port=4
  Gyro : Outport  Port=5
  wires:
  Selector/1 -> Quaternion/1
  Selector1/1 -> Position/1
  "  "/1 -> Velocity/1
  Selector2/1 -> Gyro/1
  Selector3/1 -> Sum1/1
  Sum1/1 -> Accel/1
  Constant/1 -> Sum1/2
  In1/1 -> Selector1/1, Selector/1, Selector2/1, "  "/1
  In2/1 -> Selector3/1

== matlab function SimulationLoopNew/Plant Simulation/Sensor Models/Rotate1 ==
  data: Inertial input; Body output; q input
function Body = Rotate(Inertial, q)
Body = quatRot(q) * (Inertial + 0.05 * ones(3,1));

== matlab function SimulationLoopNew/Plant Simulation/Sensor Models/MATLAB Function ==
  data: PosVel input; Rate input; GPS_RTK output; t input
function GPS_RTK = GPS(PosVel, Rate, t)

GPS_RTK = GPS_Sim(PosVel, Rate, t);

== matlab function SimulationLoopNew/Plant Simulation/Sensor Models/MATLAB Function1 ==
  data: GPS input; t input; Input input; constantsASTRA input; Accel input; z output; Gyros input; Mag input; GND input
function z = SensorFrequency(GPS, t, Input, constantsASTRA, Accel, Gyros, Mag, GND)

%z = SensorRates(Accel, Gyros, Mag, GPS, constantsASTRA, t);
%% Add Thrust Varying Oscillation
persistent phase lastT
if isempty(phase)
    phase = 0;
    lastT = 0;
end
dt = t - lastT;
lastT = t;

% Thrust vibration generator
Track = [1.3525    42.6278];
THRUST = Input(3) / constantsASTRA.MaxT * 100;
w = 2 * pi * (Track(1) * THRUST + Track(2) + 1 * randn());
phase = phase + w * dt;
MaxAmplAccel = 7;
MaxAmplGyro = 0.2;
Accel = Accel + MaxAmplAccel * THRUST / 100 * sin(phase) * (1 - GND);
Gyros = Gyros + MaxAmplGyro * THRUST / 100 * sin(phase) * (1 - GND);
z = [Accel; Gyros; Mag; GPS];

== matlab function SimulationLoopNew/Plant Simulation/Disturbance Models and Integrator/Wind/GMP Model ==
  data: t input; GMP_out output; covar input
function GMP_out = GMP(t, covar)

persistent errorval lastTime EMA
if isempty(errorval)
    errorval = 0;
    EMA = 0;
    lastTime = 0;  % Update last timestamp
end

dT = t - lastTime;

% First order Gauss Markov Process for additional disturbance
decay = 10;
beta = exp(-dT / decay);
errorval = beta * errorval + sqrt(1 - beta^2) * covar * randn;

% EMA Step to kill High Freq. Noise
EMA = ExpMovingAvg(errorval, EMA, 0.05);
GMP_out = EMA * ones(3,1);
lastTime = t;

== matlab function SimulationLoopNew/Controller and Clamping/Controller v2 ==
  data: PosTarget input; X input; constantsASTRA input; U output; T input; TRG output
function [U, TRG] = ControlFCN(PosTarget, X, constantsASTRA,  T)

    [U, TRG] = ASTRAv2_Controller(PosTarget, X, constantsASTRA,  T);

== matlab function SimulationLoopNew/Plant Simulation/Vehicle Dynamics/Dynamics ==
  data: X input; XDOT output; U input; distMode input
function XDOT = Dynamics(X, U, distMode)
if distMode == 1
    XDOT = disturbedDynamics(X, U);
else
    XDOT = nominalDynamics(X, U);
end

== matlab function SimulationLoopNew/State Estimator /Adaptive Notch Filter [ANF]/ANF Filter ==
  data: Y input; Y_FILT output; GND input; U input; IMU_Rate input; dT output
function [Y_FILT, dT] = ANF_Filter(Y, GND, U, IMU_Rate)

% Extract IMU
IMU = Y(1:9);
dT = 1 / IMU_Rate;

% Thrust PCT
THRUST = U(3) / (1.697 * 9.80145) * 100;

% ANF Filter
ANF_IMU = DigitalNF(IMU, GND, THRUST, dT);

% Combine (FILTER CURRENTLY OFF)
Y_FILT = [ANF_IMU; Y(10:15)];

== matlab function SimulationLoopNew/Controller and Clamping/Quaternion to Euler/Quaternion to Euler ==
  data: X input; Angles output
function Angles = q2eul(X)

% Complete quaternion
q = X(1:4);

% Quaternion to Euler Angles
Roll = atan2(2*(q(1) * q(2) + q(3) * q(4)), 1 - 2*(q(2)^2 + q(3)^2));
Pitch = asin(2*(q(1) * q(3) - q(4) * q(2)));
Yaw = atan2(2*(q(1) * q(4) + q(2) * q(3)), 1 - 2*(q(3)^2 + q(4)^2));

% Angle Vector
Angles = [Roll; Pitch; Yaw] * 180/pi;

== matlab function SimulationLoopNew/Controller and Clamping/Input Clamping and Rate Limiter ==
  data: U input; U output; T input
function U = INPUTFCN(U, T)

    U = inputfcn3(U, T)';

== matlab function SimulationLoopNew/Trajectory/MATLAB Function1 ==
  data: t input; Check input; X input; REF output; TRG output; ERR output
function [REF, TRG, ERR] = RefSignal(t, Check, X)

Checkpoints = Check(1:3, :);
HoldReqs = Check(4, :);
[REF, TRG, ERR] = ref_generator3(X, t, Checkpoints, HoldReqs);

== matlab function SimulationLoopNew/Plant Simulation/Sensor Models/Rotate ==
  data: Inertial input; Body output; q input
function Body = Rotate(Inertial, q)
Body = quatRot(q) * Inertial;

== matlab function SimulationLoopNew/State Estimator /Multiplicative Extended Kalman Filter [M-EKF]/Kalman Filter ==
  data: X input; Y input; GND input; X output; T input; ASTRAv2 input
function X = MEKF(X, Y, GND, T, ASTRAv2)

    % Measure simulation timestep
    persistent dt lastT lastP
    if isempty(dt)
        dt = 0;
        lastT = 0;
        lastP = eye(18);
    end
    dt = T - lastT;
    lastT = T;
    
    if GND
        [X, lastP] = GroundEstimator(X, ASTRAv2, Y, dt);
    else
        X = FlightEstimator(X, ASTRAv2, Y, dt, lastP(1:9, 1:9));
    end
end
    %X = EstimateStateFCN(X, ASTRAv2, Y, dt, GND);

== matlab function SimulationLoopNew/Plant Simulation/Disturbance Models and Integrator/Wind/MATLAB Function ==
  data: constants input; wind_vel input; X input; wind_disturb output
function wind_disturb = wind_sim(constants, wind_vel, X)

wind_disturb = wind(constants, wind_vel, X);

== matlab function SimulationLoopNew/Plant Simulation/Actuator Models/MATLAB Function ==
  data: U input; UDOT output; U_TRG input; GND input
function UDOT = Actuators(U, U_TRG, GND)

    UDOT = ActuatorDynamics(U, U_TRG, GND);
end

== matlab function SimulationLoopNew/Quaternion to Euler/Quaternion to Euler ==
  data: X input; Angles output
function Angles = q2eul(X)

% Complete quaternion
q = X(1:4);

% Quaternion to Euler Angles
Roll = atan2(2*(q(1) * q(2) + q(3) * q(4)), 1 - 2*(q(2)^2 + q(3)^2));
Pitch = asin(2*(q(1) * q(3) - q(4) * q(2)));
Yaw = atan2(2*(q(1) * q(4) + q(2) * q(3)), 1 - 2*(q(3)^2 + q(4)^2));

% Angle Vector
Angles = [Roll; Pitch; Yaw] * 180/pi;

== matlab function SimulationLoopNew/State Estimator /State Augmentator/MATLAB Function ==
  data: XKF input; X output; Y input
function X = StateAUG(XKF, Y)

% Change Filter State to Controls State
X = [XKF(1:4); XKF(5:7); XKF(8:10); Y(4:6) - XKF(11:13); XKF(11:13)];

== matlab function SimulationLoopNew/Plant Simulation/Disturbance Models and Integrator/Normalize Quaternion ==
  data: X input; X_N output
function X_N = fcn(X)
X_N = [X(1:4) / norm(X(1:4)); X(5:end)];
